simulink model "SSRP_A"  (R2023a)
settings: Solver=FixedStepDiscrete  StartTime=0.0  StopTime=inf  RelTol=1e-3
undefined symbols (not defined in the file): DiscIntNeverNeededParam
libraries: androiduilib x14, androidcommunicationlib x4, androidsensorlib x3, androidaudiovideolib x3
settings Model: Creator=Lavanya  LastModifiedBy=Lavanya
settings OptimizationCC: EnhancedBackFolding=on  PassReuseOutputArgsAs=Individual arguments  ZeroExternalMemoryAtStartup=off  ZeroInternalMemoryAtStartup=off  MaxStackSize=64  OptimizeBlockOrder=speed  DifferentSizesBufferReuse=on  OptimizationCustomize=off  EfficientTunableParamExpr=on
settings DebuggingCC: ParameterTunabilityLossMsg=error
settings HardwareCC: ProdBitPerPointer=32  ProdBitPerSizeT=32  ProdBitPerPtrDiffT=32  ProdLargestAtomicInteger=Long  ProdLargestAtomicFloat=Double  ProdWordSize=32  ProdHWDeviceType=ARM Compatible->ARM Cortex  UseEmbeddedCoderFeatures=off  UseSimulinkCoderFeatures=off
settings SFSimCC: MATLABDynamicMemAlloc=off
settings RTWCC: Description=Embedded Coder  SystemTargetFile=ert.tlc  HardwareBoard=Android Device  TLCOptions="-aInlineSetEventsForThisBaseRateFcn=TLC_FALSE -aSuppressMultiTaskScheduler=TLC_FALSE  -aRateBasedStepFcn=0"  TemplateMakefile=ert_default_tmf  RTWVerbose=off  Toolchain=Android SDK/NDK Tools
settings CodeAppCC: ForceParamTrailComments=on  IgnoreCustomStorageClasses=off  OperatorAnnotations=on  SimulinkDataObjDesc=on  SFDataObjDesc=on  InsertBlockDesc=on
settings ERTTargetCC: SupportNonInlinedSFcns=on

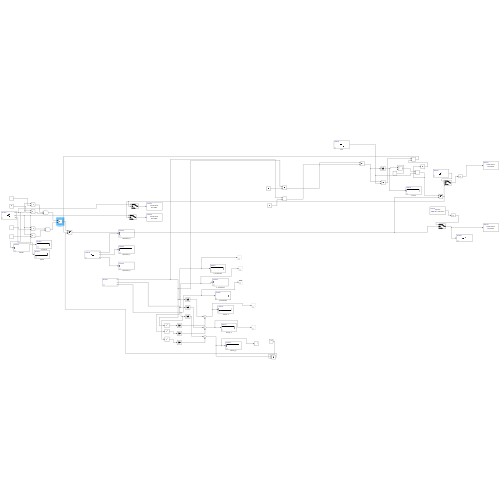
[thumbnail: Simulink's stored preview of the top-level diagram]
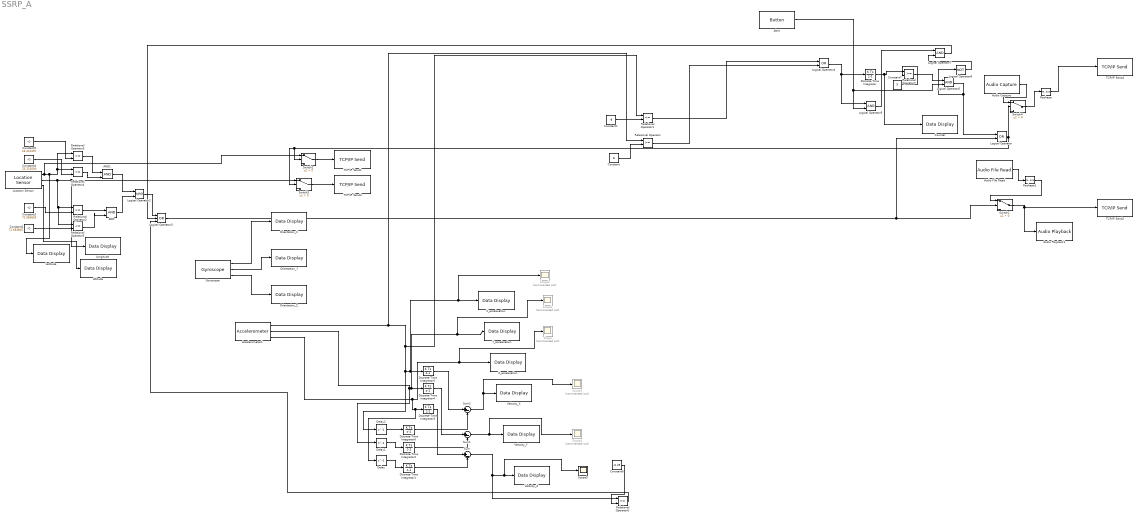
== system SSRP_A ==
  AND : Logic  IconShape=distinctive  AllPortsSameDT=off  OutDataTypeStr=boolean
  AND1 : Logic  IconShape=distinctive  AllPortsSameDT=off  OutDataTypeStr=boolean
  Accelerometer1 : androidsensorlib/Accelerometer  OutputVector=off  SampleTime=0.1  BlockPlatform=Android
  Alert : androiduilib/Button  ButtonState=Pressed  ButtonId=SSRP_A/Alert  State=on  SampleTime=0.1  BlockPlatform=Android
  Altitude : androiduilib/Data Display  DataDisplayId=SSRP_A/Altitude  Format=Float  Precision=6  SimulateUsing=Code generation  blockPlatform=Android
  Audio Capture : androidaudiovideolib/Audio Capture  SampleFreq=44100  FrameSize=4410  SampleTime=0.1  SimulateUsing=Code generation  DeviceStr=0  QueueDuration=0  BlockPlatform=Android  AudioSamplingFreq=44100
  Audio File Read : androidaudiovideolib/Audio File Read  FileName=C:\Users\Lavanya\Downloads\ssrp.wav  FrameSize=9600
  Audio Playback1 : androidaudiovideolib/Audio Playback  SampleFreq=48000  AudioSamplingFreq=48000  SampleTime=0.1  DeviceStr=0  QueueDuration=0  BlockPlatform=Android
  Constant : Constant  Value=8
  Constant1 : Constant  Value=-8
  Constant2 : Constant  Value=72.683802
  Constant3 : Constant  Value=72.683655
  Constant4 : Constant  Value=23.210500
  Constant5 : Constant  Value=23.210197
  Constant6 : Constant  Value=-0.25
  Constant7 : Constant  Value=5
  Counter : androiduilib/Data Display  DataDisplayId=SSRP_A/Counter  Format=Float  Precision=6  SimulateUsing=Code generation  blockPlatform=Android
  Delay : Delay  DelayLength=1  InitialCondition=0
  Delay1 : Delay  DelayLength=1  InitialCondition=0
  Delay2 : Delay  DelayLength=1  InitialCondition=0
  Discrete-Time Integrator{,1..6} (7 alike) : DiscreteIntegrator  SampleTime=-1  ICPrevOutput=DiscIntNeverNeededParam  ICPrevScaledInput=DiscIntNeverNeededParam
  Gyroscope : androidsensorlib/Gyroscope  OutputVector=off  SampleTime=0.1  BlockPlatform=Android
  Latitude : androiduilib/Data Display  DataDisplayId=SSRP_A/Latitude  Format=Float  Precision=6  SimulateUsing=Code generation  blockPlatform=Android
  Location Sensor : androidsensorlib/Location Sensor  OutputVector=off  SampleTime=0.1  BlockPlatform=Android
  Logical Operator : Logic  Operator=OR  AllPortsSameDT=off  OutDataTypeStr=boolean
  Logical Operator2 : Logic  Operator=NAND  AllPortsSameDT=off  OutDataTypeStr=boolean
  Logical Operator3 : Logic  Operator=OR  Inputs=3  AllPortsSameDT=off  OutDataTypeStr=boolean
  Logical Operator4 : Logic  Operator=OR  AllPortsSameDT=off  OutDataTypeStr=boolean
  Logical Operator5 : Logic  AllPortsSameDT=off  OutDataTypeStr=boolean
  Logical Operator6 : Logic  AllPortsSameDT=off  OutDataTypeStr=boolean
  Logical Operator7 : Logic  AllPortsSameDT=off  OutDataTypeStr=boolean
  Logical Operator8 : Logic  Operator=NOT  AllPortsSameDT=off  OutDataTypeStr=boolean
  Longitude : androiduilib/Data Display  DataDisplayId=SSRP_A/Longitude  Format=Float  Precision=6  SimulateUsing=Code generation  blockPlatform=Android
  Orientation_X : androiduilib/Data Display  DataDisplayId=SSRP_A/Orientation_X  Format=Float  Precision=6  SimulateUsing=Code generation  blockPlatform=Android
  Orientation_Y : androiduilib/Data Display  DataDisplayId=SSRP_A/Orientation_Y  Format=Float  Precision=6  SimulateUsing=Code generation  blockPlatform=Android
  Orientation_Z : androiduilib/Data Display  DataDisplayId=SSRP_A/Orientation_Z  Format=Float  Precision=6  SimulateUsing=Code generation  blockPlatform=Android
  Relational Operator{,2..3,6..7} (5 alike) : RelationalOperator  OutDataTypeStr=boolean  RndMeth=Simplest  InputSameDT=off
  Relational Operator1 : RelationalOperator  Operator=<=  OutDataTypeStr=boolean  RndMeth=Simplest  InputSameDT=off
  Relational Operator4 : RelationalOperator  Operator=<=  OutDataTypeStr=boolean  RndMeth=Simplest  InputSameDT=off
  Relational Operator5 : RelationalOperator  Operator=<=  OutDataTypeStr=boolean  RndMeth=Simplest  InputSameDT=off
  Reshape : Reshape  OutputDimensionality=Customize  OutputDimensions=[8820,1]
  Reshape1 : Reshape  OutputDimensionality=Customize  OutputDimensions=[4800,2]
  Scope{,1..4} (5 alike) : Scope  Commented=on
  Scope5 : Scope
  Sum : Sum  Inputs=|+-
  Sum1 : Sum  Inputs=|+-
  Sum2 : Sum  Inputs=|+-
  Switch{1..4} (4 alike) : Switch  Criteria=u2 > Threshold  SaturateOnIntegerOverflow=off  InputSameDT=off
  TCP/IP Send1 : androidcommunicationlib/TCP//IP Send  TCPSendId=SSRP_A/TCP//IP_Send1  Mode_=Server  LocalServerPort_=30001  RemoteAddr_=10.7.15.181  RemoteServerPort_=25000  ClientPortBindingSelection_=off  ClientPortToBind_=35000  BlockingMode_=off  BlockTimeout_=0.1
  TCP/IP Send2 : androidcommunicationlib/TCP//IP Send  TCPSendId=SSRP_A/TCP//IP_Send2  Mode_=Server  LocalServerPort_=25007  RemoteAddr_=10.7.15.181  RemoteServerPort_=25000  ClientPortBindingSelection_=off  ClientPortToBind_=35000  BlockingMode_=off  BlockTimeout_=0.1
  TCP/IP Send3 : androidcommunicationlib/TCP//IP Send  TCPSendId=SSRP_A/TCP//IP_Send3  Mode_=Server  LocalServerPort_=30002  RemoteAddr_=10.7.15.181  RemoteServerPort_=25000  ClientPortBindingSelection_=off  ClientPortToBind_=35000  BlockingMode_=off  BlockTimeout_=0.1
  TCP/IP Send4 : androidcommunicationlib/TCP//IP Send  TCPSendId=SSRP_A/TCP//IP_Send4  Mode_=Server  LocalServerPort_=25006  RemoteAddr_=10.7.15.181  RemoteServerPort_=25000  ClientPortBindingSelection_=off  ClientPortToBind_=35000  BlockingMode_=off  BlockTimeout_=0.1
  Velocity_X : androiduilib/Data Display  DataDisplayId=SSRP_A/Velocity_X  Format=Float  Precision=6  SimulateUsing=Code generation  blockPlatform=Android
  Velocity_Y : androiduilib/Data Display  DataDisplayId=SSRP_A/Velocity_Y  Format=Float  Precision=6  SimulateUsing=Code generation  blockPlatform=Android
  Velocity_Z : androiduilib/Data Display  DataDisplayId=SSRP_A/Velocity_Z  Format=Float  Precision=6  SimulateUsing=Code generation  blockPlatform=Android
  X_acceleration : androiduilib/Data Display  DataDisplayId=SSRP_A/X_acceleration  Format=Float  Precision=6  SimulateUsing=Code generation  blockPlatform=Android
  Y_acceleration : androiduilib/Data Display  DataDisplayId=SSRP_A/Y_acceleration  Format=Float  Precision=6  SimulateUsing=Code generation  blockPlatform=Android
  Z_acceleration : androiduilib/Data Display  DataDisplayId=SSRP_A/Z_acceleration  Format=Float  Precision=6  SimulateUsing=Code generation  blockPlatform=Android
  wires:
  Constant/1 -> Relational Operator/2
  Constant1/1 -> Relational Operator1/2
  Sum1/1 -> Scope4/1, Velocity_Y/1
  Discrete-Time Integrator3/1 -> Sum/1
  Delay1/1 -> Discrete-Time Integrator2/1
  Discrete-Time Integrator4/1 -> Sum1/1
  Discrete-Time Integrator5/1 -> Sum2/1
  Delay2/1 -> Discrete-Time Integrator6/1
  Sum/1 -> Relational Operator6/1, Scope5/1, Velocity_Z/1
  Accelerometer1/1 -> Relational Operator/1, Relational Operator1/1, Delay2/1, Scope2/1, X_acceleration/1, Discrete-Time Integrator5/1
  Discrete-Time Integrator2/1 -> Sum1/2
  Accelerometer1/3 -> Scope/1, Z_acceleration/1, Delay/1, Discrete-Time Integrator3/1
  Delay/1 -> Discrete-Time Integrator1/1
  Accelerometer1/2 -> Discrete-Time Integrator4/1, Scope1/1, Y_acceleration/1, Delay1/1
  Discrete-Time Integrator6/1 -> Sum2/2
  Sum2/1 -> Scope3/1, Velocity_X/1
  Discrete-Time Integrator1/1 -> Sum/2
  AND/1 -> Logical Operator2/2
  Constant5/1 -> Relational Operator3/2
  Relational Operator5/1 -> AND/2
  Switch1/1 -> Audio Playback1/1, TCP/IP Send2/1
  Constant2/1 -> Relational Operator5/2
  Constant3/1 -> Relational Operator2/2
  Reshape1/1 -> Switch1/1
  Location Sensor/3 -> Altitude/1
  Constant4/1 -> Relational Operator4/2
  Audio File Read/1 -> Reshape1/1
  Relational Operator4/1 -> AND1/2
  Relational Operator3/1 -> AND1/1
  AND1/1 -> Logical Operator2/1
  Location Sensor/1 -> Switch2/1, Latitude/1, Relational Operator4/1, Relational Operator3/1
  Location Sensor/2 -> Longitude/1, Switch3/1, Relational Operator5/1, Relational Operator2/1
  Relational Operator2/1 -> AND/1
  Logical Operator2/1 -> Logical Operator3/1
  Logical Operator3/1 -> Logical Operator/2, Switch1/2
  Relational Operator6/1 -> Logical Operator3/3
  Switch3/1 -> TCP/IP Send3/1
  Switch2/1 -> TCP/IP Send1/1
  Switch4/1 -> Reshape/1
  Discrete-Time Integrator/1 -> Counter/1, Relational Operator7/1
  Constant7/1 -> Relational Operator7/2
  Audio Capture/1 -> Switch4/1
  Reshape/1 -> TCP/IP Send4/1
  Logical Operator5/1 -> Logical Operator7/1
  Relational Operator7/1 -> Logical Operator6/1
  Logical Operator8/1 -> Logical Operator7/2
  Alert/1 -> Logical Operator6/2, Logical Operator5/2
  Relational Operator/1 -> Logical Operator4/2
  Relational Operator1/1 -> Logical Operator4/1
  Logical Operator6/1 -> Logical Operator8/1, Logical Operator/1
  Logical Operator4/1 -> Logical Operator5/1, Discrete-Time Integrator/1
  Logical Operator7/1 -> Logical Operator3/2
  Gyroscope/1 -> Orientation_X/1
  Gyroscope/2 -> Orientation_Y/1
  Gyroscope/3 -> Orientation_Z/1
  Constant6/1 -> Relational Operator6/2
  Logical Operator/1 -> Switch3/2, Switch2/2, Switch4/2
